simulink model "quad_control"  (Simulink 10.0)
settings: Solver=ode45  StartTime=0.0  StopTime=20  RelTol=1e-3  EnableMultiTasking=on
undefined symbols (not defined in the file): X, x, Y, Z
libraries: sm_lib x84, nesl_utility x46, simulink x30, fl_lib x4, sm_double_wishbone_suspension_lib x2, aerolibtransform2 x2, vrlib x1
(part 1 of 3)
settings Model: Creator=abdkadma  LastModifiedBy=bhisma
settings DataIOCC: LimitDataPoints=on
settings DebuggingCC: UnderspecifiedInitializationDetection=Simplified  MergeDetectMultiDrivingBlocksExec=error  SolverPrmCheckMsg=warning
settings GRTTargetCC: GeneratePreprocessorConditionals=Disable all  CombineOutputUpdateFcns=on  GRTInterface=off
settings ConfigComp: CovExternalEMLEnable=off
settings SimscapeCC: SimscapeNormalizeSystem=off
settings ConfigurationSet: Description=SimMechanics 2G

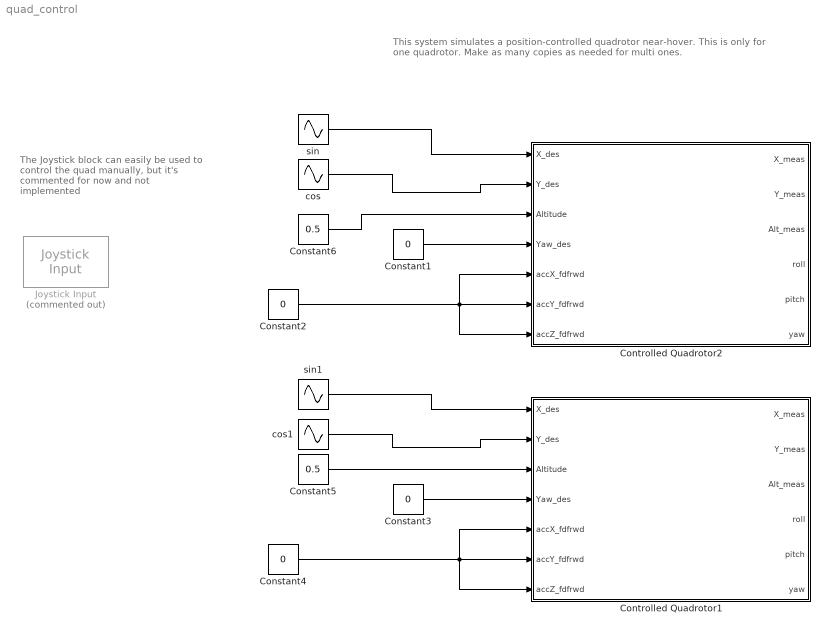
== system quad_control ==
  note: The Joystick block can easily
      | be used to control the quad manually,
      | but it's commented for now and
      | not implemented
  note: This system simulates a position-controlled quadrotor
      | near-hover. This is only for one quadrotor. Make as many copies as needed
      | for multi ones.
  Constant{1..4} (4 alike) : Constant  Value=0
  Constant5 : Constant  Value=0.5
  Constant6 : Constant  Value=0.5
  Controlled Quadrotor1 : Subsystem
      mask Display:
      | image('quadPic.jpg')
      | port_label('input',1,'x_des')
      | port_label('input',2,'y_des')
      | port_label('input',3,'Alt_des')
      | port_label('input',4,'Yaw_des')
      | port_label('input',5,'AccX_fedFwd')
      | port_label('input',6,'AccY_fedFwd')
      | port_label('input',7,'AccZ_fedFwd')
      | 
      | port_label('output',1,'x_meas')
      | port_label('output',2,'y_meas')
      | port_label('output',3,'z_meas')
      | port_label('output',4,'roll_meas')
      | port_label('output',5,'pitch_meas')
      | port_label('output',6,'yaw_meas')
  Controlled Quadrotor2 : Subsystem
      mask Display:
      | image('quadPic.jpg')
      | port_label('input',1,'x_des')
      | port_label('input',2,'y_des')
      | port_label('input',3,'Alt_des')
      | port_label('input',4,'Yaw_des')
      | port_label('input',5,'AccX_fedFwd')
      | port_label('input',6,'AccY_fedFwd')
      | port_label('input',7,'AccZ_fedFwd')
      | 
      | port_label('output',1,'x_meas')
      | port_label('output',2,'y_meas')
      | port_label('output',3,'z_meas')
      | port_label('output',4,'roll_meas')
      | port_label('output',5,'pitch_meas')
      | port_label('output',6,'yaw_meas')
  Joystick Input : vrlib/Joystick Input  Commented=on  joyid=1  adjustports=on  forcefeed=off
      settings: SourceProductName=Simulink
  cos : Sin  Amplitude=2  Phase=pi/2  SampleTime=0
  cos1 : Sin  SampleTime=0
  sin : Sin  Amplitude=2  SampleTime=0
  sin1 : Sin  Phase=pi/2  SampleTime=0
  wires:
  sin/1 -> Controlled Quadrotor2/1(X_des)
  cos/1 -> Controlled Quadrotor2/2(Y_des)
  Constant1/1 -> Controlled Quadrotor2/4(Yaw_des)
  Constant2/1 -> Controlled Quadrotor2/7(accZ_fdfrwd), Controlled Quadrotor2/5(accX_fdfrwd), Controlled Quadrotor2/6(accY_fdfrwd)
  Constant6/1 -> Controlled Quadrotor2/3(Altitude)
  sin1/1 -> Controlled Quadrotor1/1(X_des)
  cos1/1 -> Controlled Quadrotor1/2(Y_des)
  Constant3/1 -> Controlled Quadrotor1/4(Yaw_des)
  Constant4/1 -> Controlled Quadrotor1/7(accZ_fdfrwd), Controlled Quadrotor1/5(accX_fdfrwd), Controlled Quadrotor1/6(accY_fdfrwd)
  Constant5/1 -> Controlled Quadrotor1/3(Altitude)

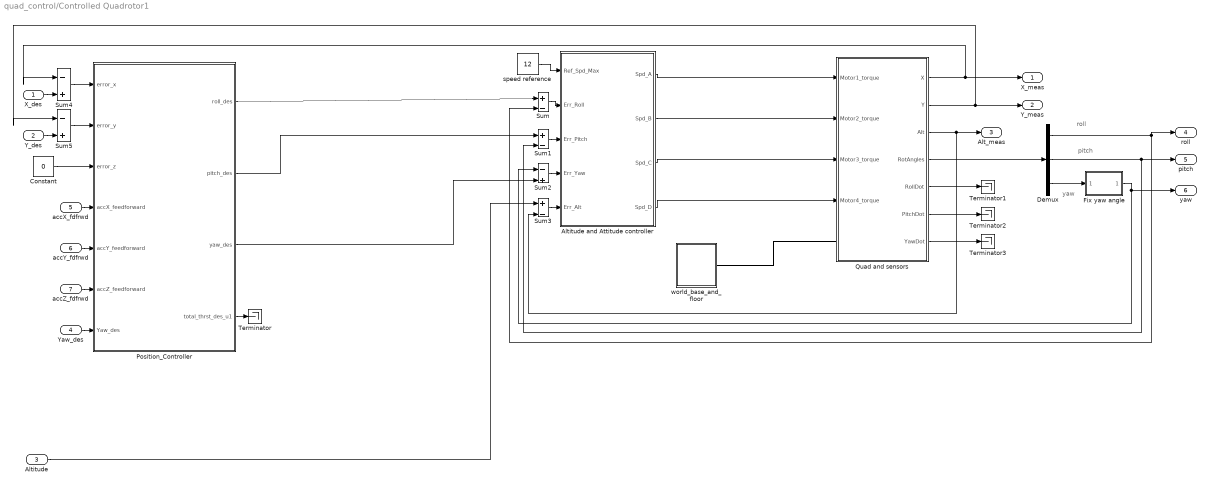
== system quad_control/Controlled Quadrotor1 ==
  note: yaw
  note: pitch
  note: roll
  X_des : Inport
  Y_des : Inport  Port=2
  Altitude : Inport  Port=3
  Yaw_des : Inport  Port=4
  accX_fdfrwd : Inport  Port=5
  accY_fdfrwd : Inport  Port=6
  accZ_fdfrwd : Inport  Port=7
  Altitude and Attitude controller : Subsystem
  Constant : Constant  Value=0
  Demux : Demux  Outputs=3
  Fix yaw angle : MATLAB Function  TreatAsAtomicUnit=on
  Position_Controller : Subsystem
  Quad and sensors : Subsystem
  Sum : Sum  Inputs=|+-
  Sum1 : Sum  Inputs=|+-
  Sum2 : Sum  Inputs=|-+
  Sum3 : Sum  Inputs=|+-
  Sum4 : Sum  Inputs=|-+
  Sum5 : Sum  Inputs=|-+
  Terminator{,1..3} (4 alike) : Terminator
  speed reference : Constant  Value=12
  world_base_and_floor : Subsystem
  X_meas : Outport
  Y_meas : Outport  Port=2
  Alt_meas : Outport  Port=3
  roll : Outport  Port=4
  pitch : Outport  Port=5
  yaw : Outport  Port=6
  wires:
  speed reference/1 -> Altitude and Attitude controller/1(Ref_Spd_Max)
  Sum1/1 -> Altitude and Attitude controller/3(Err_Pitch)
  Sum2/1 -> Altitude and Attitude controller/4(Err_Yaw)
  Sum3/1 -> Altitude and Attitude controller/5(Err_Alt)
  Altitude and Attitude controller/3(Spd_C) -> Quad and sensors/3(Motor3_torque)
  Altitude and Attitude controller/2(Spd_B) -> Quad and sensors/2(Motor2_torque)
  Altitude and Attitude controller/4(Spd_D) -> Quad and sensors/4(Motor4_torque)
  Altitude and Attitude controller/1(Spd_A) -> Quad and sensors/1(Motor1_torque)
  Demux/3 -> Fix yaw angle/1(yawangle)
  Position_Controller/3(yaw_des) -> Sum2/2
  Sum4/1 -> Position_Controller/1(error_x)
  Sum5/1 -> Position_Controller/2(error_y)
  Quad and sensors/1(X) -> X_meas/1, Sum4/1
  Position_Controller/1(roll_des) -> Sum/1
  Position_Controller/2(pitch_des) -> Sum1/1
  Sum/1 -> Altitude and Attitude controller/2(Err_Roll)
  accZ_fdfrwd/1 -> Position_Controller/6(accZ_feedforward)
  X_des/1 -> Sum4/2
  Altitude/1 -> Sum3/1
  Y_des/1 -> Sum5/2
  accY_fdfrwd/1 -> Position_Controller/5(accY_feedforward)
  accX_fdfrwd/1 -> Position_Controller/4(accX_feedforward)
  Position_Controller/4(total_thrst_des_u1) -> Terminator/1
  Constant/1 -> Position_Controller/3(error_z)
  Quad and sensors/5(RollDot) -> Terminator1/1
  Yaw_des/1 -> Position_Controller/7(Yaw_des)
  Quad and sensors/2(Y) -> Y_meas/1, Sum5/1
  Quad and sensors/3(Alt) -> Alt_meas/1, Sum3/2
  Quad and sensors/6(PitchDot) -> Terminator2/1
  Quad and sensors/7(YawDot) -> Terminator3/1
  Quad and sensors/4(RotAngles) -> Demux/1
  Fix yaw angle/1(anglefix) -> yaw/1, Sum2/1
  Demux/2 -> pitch/1, Sum1/2
  Demux/1 -> Sum/2, roll/1
  connections:
  world_base_and_floor/RConn1 -- Quad and sensors/LConn1

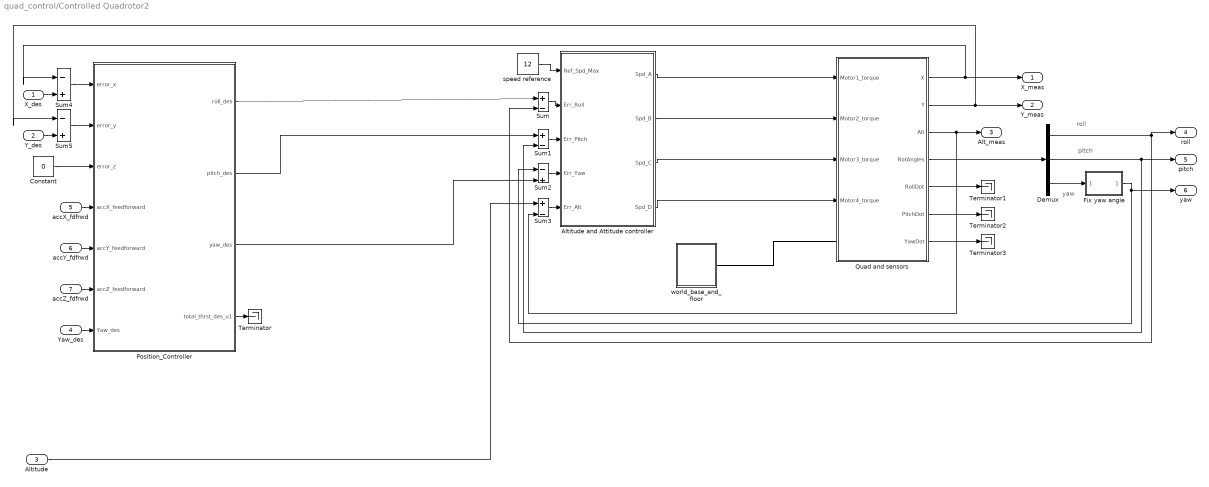
== system quad_control/Controlled Quadrotor2 ==
  note: yaw
  note: pitch
  note: roll
  X_des : Inport
  Y_des : Inport  Port=2
  Altitude : Inport  Port=3
  Yaw_des : Inport  Port=4
  accX_fdfrwd : Inport  Port=5
  accY_fdfrwd : Inport  Port=6
  accZ_fdfrwd : Inport  Port=7
  Altitude and Attitude controller : Subsystem
  Constant : Constant  Value=0
  Demux : Demux  Outputs=3
  Fix yaw angle : MATLAB Function  TreatAsAtomicUnit=on
  Position_Controller : Subsystem
  Quad and sensors : Subsystem
  Sum : Sum  Inputs=|+-
  Sum1 : Sum  Inputs=|+-
  Sum2 : Sum  Inputs=|-+
  Sum3 : Sum  Inputs=|+-
  Sum4 : Sum  Inputs=|-+
  Sum5 : Sum  Inputs=|-+
  Terminator{,1..3} (4 alike) : Terminator
  speed reference : Constant  Value=12
  world_base_and_floor : Subsystem
  X_meas : Outport
  Y_meas : Outport  Port=2
  Alt_meas : Outport  Port=3
  roll : Outport  Port=4
  pitch : Outport  Port=5
  yaw : Outport  Port=6
  wires:
  speed reference/1 -> Altitude and Attitude controller/1(Ref_Spd_Max)
  Sum1/1 -> Altitude and Attitude controller/3(Err_Pitch)
  Sum2/1 -> Altitude and Attitude controller/4(Err_Yaw)
  Sum3/1 -> Altitude and Attitude controller/5(Err_Alt)
  Altitude and Attitude controller/3(Spd_C) -> Quad and sensors/3(Motor3_torque)
  Altitude and Attitude controller/2(Spd_B) -> Quad and sensors/2(Motor2_torque)
  Altitude and Attitude controller/4(Spd_D) -> Quad and sensors/4(Motor4_torque)
  Altitude and Attitude controller/1(Spd_A) -> Quad and sensors/1(Motor1_torque)
  Demux/3 -> Fix yaw angle/1(yawangle)
  Position_Controller/3(yaw_des) -> Sum2/2
  Sum4/1 -> Position_Controller/1(error_x)
  Sum5/1 -> Position_Controller/2(error_y)
  Quad and sensors/1(X) -> X_meas/1, Sum4/1
  Position_Controller/1(roll_des) -> Sum/1
  Position_Controller/2(pitch_des) -> Sum1/1
  Sum/1 -> Altitude and Attitude controller/2(Err_Roll)
  accZ_fdfrwd/1 -> Position_Controller/6(accZ_feedforward)
  X_des/1 -> Sum4/2
  Altitude/1 -> Sum3/1
  Y_des/1 -> Sum5/2
  accY_fdfrwd/1 -> Position_Controller/5(accY_feedforward)
  accX_fdfrwd/1 -> Position_Controller/4(accX_feedforward)
  Position_Controller/4(total_thrst_des_u1) -> Terminator/1
  Constant/1 -> Position_Controller/3(error_z)
  Quad and sensors/5(RollDot) -> Terminator1/1
  Yaw_des/1 -> Position_Controller/7(Yaw_des)
  Quad and sensors/2(Y) -> Y_meas/1, Sum5/1
  Quad and sensors/3(Alt) -> Alt_meas/1, Sum3/2
  Quad and sensors/6(PitchDot) -> Terminator2/1
  Quad and sensors/7(YawDot) -> Terminator3/1
  Quad and sensors/4(RotAngles) -> Demux/1
  Fix yaw angle/1(anglefix) -> yaw/1, Sum2/1
  Demux/2 -> pitch/1, Sum1/2
  Demux/1 -> Sum/2, roll/1
  connections:
  world_base_and_floor/RConn1 -- Quad and sensors/LConn1

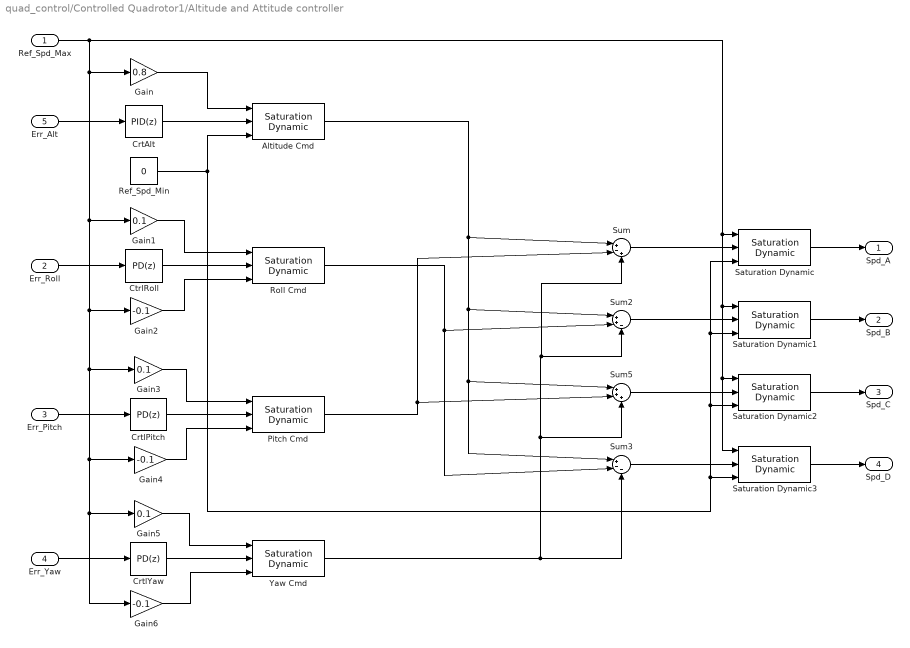
== system quad_control/Controlled Quadrotor1/Altitude and Attitude controller ==
  Ref_Spd_Max : Inport
  Err_Roll : Inport  Port=2
  Err_Pitch : Inport  Port=3
  Err_Yaw : Inport  Port=4
  Err_Alt : Inport  Port=5
  Altitude Cmd : simulink/Discontinuities/Saturation Dynamic  OutMin=[]  OutMax=[]  OutDataTypeStr=Inherit: Same as second input  OutDataType=fixdt(1, 16)  OutScaling=2^-10  DoSatur=off
  CrtAlt : simulink/Continuous/PID Controller  Controller=PID  TimeDomain=Discrete-time  SampleTime=0.001  IntegratorMethod=Forward Euler  FilterMethod=Forward Euler  Form=Parallel  P=20  I=10  D=5  N=100  InitialConditionSource=internal  InitialConditionForIntegrator=0  InitialConditionForFilter=0  ExternalReset=none  LimitOutput=off  UpperSaturationLimit=0.116  LowerSaturationLimit=-0.116  LinearizeAsGain=off  AntiWindupMode=none  Kb=1  TrackingMode=off  Kt=1  PParamMin=[]  PParamMax=[]  IParamMin=[]  IParamMax=[]  DParamMin=[]  DParamMax=[]  NParamMin=[]  NParamMax=[]  KbParamMin=[]  KbParamMax=[]  KtParamMin=[]  KtParamMax=[]  POutMin=[]  POutMax=[]  IOutMin=[]  IOutMax=[]  DOutMin=[]  DOutMax=[]  NOutMin=[]  NOutMax=[]  KbOutMin=[]  KbOutMax=[]  KtOutMin=[]  KtOutMax=[]  IntegratorOutMin=[]  IntegratorOutMax=[]  FilterOutMin=[]  FilterOutMax=[]  SumOutMin=[]  SumOutMax=[]  SumI1OutMin=[]  SumI1OutMax=[]  SumI2OutMin=[]  SumI2OutMax=[]  SumI3OutMin=[]  SumI3OutMax=[]  SumDOutMin=[]  SumDOutMax=[]  SaturationOutMin=[]  SaturationOutMax=[]  IntegratorContinuousStateAttributes=''  IntegratorStateMustResolveToSignalObject=off  IntegratorRTWStateStorageClass=Auto  FilterContinuousStateAttributes=''  FilterStateMustResolveToSignalObject=off  FilterRTWStateStorageClass=Auto  DifferentiatorICPrevScaledInput=0  DifferentiatorOutMin=[]  DifferentiatorOutMax=[]  UseFilter=on
  CrtlPitch : simulink/Continuous/PID Controller  Controller=PD  TimeDomain=Discrete-time  SampleTime=0.001  IntegratorMethod=Forward Euler  FilterMethod=Forward Euler  Form=Parallel  P=2  I=0  D=1  N=100  InitialConditionSource=internal  InitialConditionForIntegrator=0  InitialConditionForFilter=0  ExternalReset=none  LimitOutput=off  UpperSaturationLimit=+Inf  LowerSaturationLimit=0  LinearizeAsGain=off  AntiWindupMode=none  Kb=1  TrackingMode=off  Kt=1  PParamMin=[]  PParamMax=[]  IParamMin=[]  IParamMax=[]  DParamMin=[]  DParamMax=[]  NParamMin=[]  NParamMax=[]  KbParamMin=[]  KbParamMax=[]  KtParamMin=[]  KtParamMax=[]  POutMin=[]  POutMax=[]  IOutMin=[]  IOutMax=[]  DOutMin=[]  DOutMax=[]  NOutMin=[]  NOutMax=[]  KbOutMin=[]  KbOutMax=[]  KtOutMin=[]  KtOutMax=[]  IntegratorOutMin=[]  IntegratorOutMax=[]  FilterOutMin=[]  FilterOutMax=[]  SumOutMin=[]  SumOutMax=[]  SumI1OutMin=[]  SumI1OutMax=[]  SumI2OutMin=[]  SumI2OutMax=[]  SumI3OutMin=[]  SumI3OutMax=[]  SumDOutMin=[]  SumDOutMax=[]  SaturationOutMin=[]  SaturationOutMax=[]  IntegratorContinuousStateAttributes=''  IntegratorStateMustResolveToSignalObject=off  IntegratorRTWStateStorageClass=Auto  FilterContinuousStateAttributes=''  FilterStateMustResolveToSignalObject=off  FilterRTWStateStorageClass=Auto  DifferentiatorICPrevScaledInput=0  DifferentiatorOutMin=[]  DifferentiatorOutMax=[]  UseFilter=on
  CrtlYaw : simulink/Continuous/PID Controller  Controller=PD  TimeDomain=Discrete-time  SampleTime=0.001  IntegratorMethod=Forward Euler  FilterMethod=Forward Euler  Form=Parallel  P=0.05  I=1  D=0.01  N=100  InitialConditionSource=internal  InitialConditionForIntegrator=0  InitialConditionForFilter=0  ExternalReset=none  LimitOutput=off  UpperSaturationLimit=0.01  LowerSaturationLimit=-0.01  LinearizeAsGain=off  AntiWindupMode=none  Kb=1  TrackingMode=off  Kt=1  PParamMin=[]  PParamMax=[]  IParamMin=[]  IParamMax=[]  DParamMin=[]  DParamMax=[]  NParamMin=[]  NParamMax=[]  KbParamMin=[]  KbParamMax=[]  KtParamMin=[]  KtParamMax=[]  POutMin=[]  POutMax=[]  IOutMin=[]  IOutMax=[]  DOutMin=[]  DOutMax=[]  NOutMin=[]  NOutMax=[]  KbOutMin=[]  KbOutMax=[]  KtOutMin=[]  KtOutMax=[]  IntegratorOutMin=[]  IntegratorOutMax=[]  FilterOutMin=[]  FilterOutMax=[]  SumOutMin=[]  SumOutMax=[]  SumI1OutMin=[]  SumI1OutMax=[]  SumI2OutMin=[]  SumI2OutMax=[]  SumI3OutMin=[]  SumI3OutMax=[]  SumDOutMin=[]  SumDOutMax=[]  SaturationOutMin=[]  SaturationOutMax=[]  IntegratorContinuousStateAttributes=''  IntegratorStateMustResolveToSignalObject=off  IntegratorRTWStateStorageClass=Auto  FilterContinuousStateAttributes=''  FilterStateMustResolveToSignalObject=off  FilterRTWStateStorageClass=Auto  DifferentiatorICPrevScaledInput=0  DifferentiatorOutMin=[]  DifferentiatorOutMax=[]  UseFilter=on
  CtrlRoll : simulink/Continuous/PID Controller  Controller=PD  TimeDomain=Discrete-time  SampleTime=0.001  IntegratorMethod=Forward Euler  FilterMethod=Forward Euler  Form=Parallel  P=2  I=0  D=1  N=100  InitialConditionSource=internal  InitialConditionForIntegrator=0  InitialConditionForFilter=0  ExternalReset=none  LimitOutput=off  UpperSaturationLimit=+Inf  LowerSaturationLimit=0  LinearizeAsGain=off  AntiWindupMode=none  Kb=1  TrackingMode=off  Kt=1  PParamMin=[]  PParamMax=[]  IParamMin=[]  IParamMax=[]  DParamMin=[]  DParamMax=[]  NParamMin=[]  NParamMax=[]  KbParamMin=[]  KbParamMax=[]  KtParamMin=[]  KtParamMax=[]  POutMin=[]  POutMax=[]  IOutMin=[]  IOutMax=[]  DOutMin=[]  DOutMax=[]  NOutMin=[]  NOutMax=[]  KbOutMin=[]  KbOutMax=[]  KtOutMin=[]  KtOutMax=[]  IntegratorOutMin=[]  IntegratorOutMax=[]  FilterOutMin=[]  FilterOutMax=[]  SumOutMin=[]  SumOutMax=[]  SumI1OutMin=[]  SumI1OutMax=[]  SumI2OutMin=[]  SumI2OutMax=[]  SumI3OutMin=[]  SumI3OutMax=[]  SumDOutMin=[]  SumDOutMax=[]  SaturationOutMin=[]  SaturationOutMax=[]  IntegratorContinuousStateAttributes=''  IntegratorStateMustResolveToSignalObject=off  IntegratorRTWStateStorageClass=Auto  FilterContinuousStateAttributes=''  FilterStateMustResolveToSignalObject=off  FilterRTWStateStorageClass=Auto  DifferentiatorICPrevScaledInput=0  DifferentiatorOutMin=[]  DifferentiatorOutMax=[]  UseFilter=on
  Gain : Gain  Gain=0.8
  Gain1 : Gain  Gain=0.1
  Gain2 : Gain  Gain=-0.1
  Gain3 : Gain  Gain=0.1
  Gain4 : Gain  Gain=-0.1
  Gain5 : Gain  Gain=0.1
  Gain6 : Gain  Gain=-0.1
  Pitch Cmd : simulink/Discontinuities/Saturation Dynamic  OutMin=[]  OutMax=[]  OutDataTypeStr=Inherit: Same as second input  OutDataType=fixdt(1, 16)  OutScaling=2^-10  DoSatur=off
      settings: LockScale=on
  Ref_Spd_Min : Constant  Value=0
  Roll Cmd : simulink/Discontinuities/Saturation Dynamic  OutMin=[]  OutMax=[]  OutDataTypeStr=Inherit: Same as second input  OutDataType=fixdt(1, 16)  OutScaling=2^-10  DoSatur=off
      settings: LockScale=on
  Saturation Dynamic{,1..3} (4 alike) : simulink/Discontinuities/Saturation Dynamic  OutMin=[]  OutMax=[]  OutDataTypeStr=Inherit: Same as second input  OutDataType=fixdt(1, 16)  OutScaling=2^-10  DoSatur=off
  Sum : Sum  Inputs=|+-+
  Sum2 : Sum  Inputs=|++-
  Sum3 : Sum  Inputs=|+--
  Sum5 : Sum  Inputs=|+++
  Yaw Cmd : simulink/Discontinuities/Saturation Dynamic  OutMin=[]  OutMax=[]  OutDataTypeStr=Inherit: Same as second input  OutDataType=fixdt(1, 16)  OutScaling=2^-10  DoSatur=off
      settings: LockScale=on
  Spd_A : Outport
  Spd_B : Outport  Port=2
  Spd_C : Outport  Port=3
  Spd_D : Outport  Port=4
  wires:
  Saturation Dynamic/1 -> Spd_A/1
  Saturation Dynamic1/1 -> Spd_B/1
  Saturation Dynamic2/1 -> Spd_C/1
  Saturation Dynamic3/1 -> Spd_D/1
  Sum/1 -> Saturation Dynamic/2
  Sum2/1 -> Saturation Dynamic1/2
  Sum5/1 -> Saturation Dynamic2/2
  Sum3/1 -> Saturation Dynamic3/2
  Ref_Spd_Max/1 -> Gain3/1, Gain4/1, Gain5/1, Gain6/1, Gain2/1, Gain1/1, Gain/1, Saturation Dynamic3/1, Saturation Dynamic2/1, Saturation Dynamic1/1, Saturation Dynamic/1
  Ref_Spd_Min/1 -> Saturation Dynamic/3, Saturation Dynamic1/3, Saturation Dynamic2/3, Saturation Dynamic3/3, Altitude Cmd/3
  Err_Alt/1 -> CrtAlt/1
  CrtAlt/1 -> Altitude Cmd/2
  Altitude Cmd/1 -> Sum3/1, Sum5/1, Sum2/1, Sum/1
  Err_Roll/1 -> CtrlRoll/1
  Gain/1 -> Altitude Cmd/1
  CtrlRoll/1 -> Roll Cmd/2
  Gain2/1 -> Roll Cmd/3
  Gain1/1 -> Roll Cmd/1
  Roll Cmd/1 -> Sum2/2, Sum3/2
  Err_Pitch/1 -> CrtlPitch/1
  CrtlPitch/1 -> Pitch Cmd/2
  Gain3/1 -> Pitch Cmd/1
  Gain4/1 -> Pitch Cmd/3
  Pitch Cmd/1 -> Sum/2, Sum5/2
  Err_Yaw/1 -> CrtlYaw/1
  CrtlYaw/1 -> Yaw Cmd/2
  Gain5/1 -> Yaw Cmd/1
  Gain6/1 -> Yaw Cmd/3
  Yaw Cmd/1 -> Sum/3, Sum2/3, Sum5/3, Sum3/3

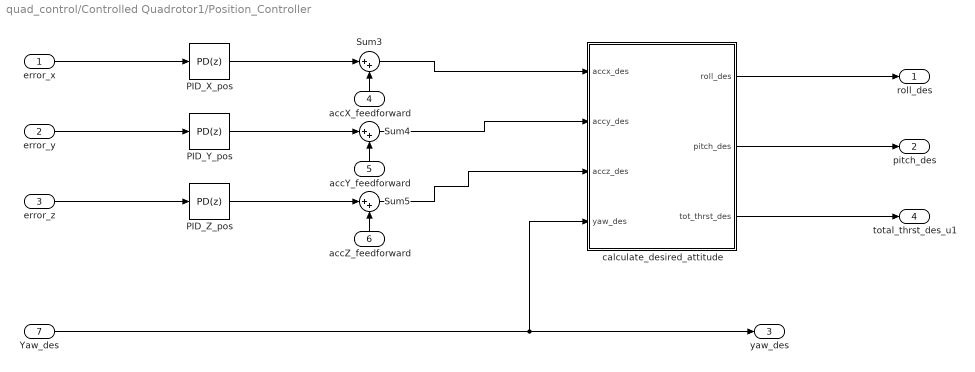
== system quad_control/Controlled Quadrotor1/Position_Controller ==
  error_x : Inport
  error_y : Inport  Port=2
  error_z : Inport  Port=3
  accX_feedforward : Inport  Port=4
  accY_feedforward : Inport  Port=5
  accZ_feedforward : Inport  Port=6
  Yaw_des : Inport  Port=7
  PID_X_pos : simulink/Continuous/PID Controller  Controller=PD  TimeDomain=Discrete-time  SampleTime=0.01  IntegratorMethod=Forward Euler  FilterMethod=Forward Euler  Form=Parallel  P=10  I=1  D=3  N=148.847847480226  InitialConditionSource=internal  InitialConditionForIntegrator=0  InitialConditionForFilter=0  ExternalReset=none  LimitOutput=off  UpperSaturationLimit=inf  LowerSaturationLimit=-inf  LinearizeAsGain=on  AntiWindupMode=none  Kb=1  TrackingMode=off  Kt=1  PParamMin=[]  PParamMax=[]  IParamMin=[]  IParamMax=[]  DParamMin=[]  DParamMax=[]  NParamMin=[]  NParamMax=[]  KbParamMin=[]  KbParamMax=[]  KtParamMin=[]  KtParamMax=[]  POutMin=[]  POutMax=[]  IOutMin=[]  IOutMax=[]  DOutMin=[]  DOutMax=[]  NOutMin=[]  NOutMax=[]  KbOutMin=[]  KbOutMax=[]  KtOutMin=[]  KtOutMax=[]  IntegratorOutMin=[]  IntegratorOutMax=[]  FilterOutMin=[]  FilterOutMax=[]  SumOutMin=[]  SumOutMax=[]  SumI1OutMin=[]  SumI1OutMax=[]  SumI2OutMin=[]  SumI2OutMax=[]  SumI3OutMin=[]  SumI3OutMax=[]  SumDOutMin=[]  SumDOutMax=[]  SaturationOutMin=[]  SaturationOutMax=[]  IntegratorContinuousStateAttributes=''  IntegratorStateMustResolveToSignalObject=off  IntegratorRTWStateStorageClass=Auto  FilterContinuousStateAttributes=''  FilterStateMustResolveToSignalObject=off  FilterRTWStateStorageClass=Auto  DifferentiatorICPrevScaledInput=0  DifferentiatorOutMin=[]  DifferentiatorOutMax=[]  UseFilter=on
  PID_Y_pos : simulink/Continuous/PID Controller  Controller=PD  TimeDomain=Discrete-time  SampleTime=0.01  IntegratorMethod=Forward Euler  FilterMethod=Forward Euler  Form=Parallel  P=10  I=1  D=3  N=100  InitialConditionSource=internal  InitialConditionForIntegrator=0  InitialConditionForFilter=0  ExternalReset=none  LimitOutput=off  UpperSaturationLimit=inf  LowerSaturationLimit=-inf  LinearizeAsGain=on  AntiWindupMode=none  Kb=1  TrackingMode=off  Kt=1  PParamMin=[]  PParamMax=[]  IParamMin=[]  IParamMax=[]  DParamMin=[]  DParamMax=[]  NParamMin=[]  NParamMax=[]  KbParamMin=[]  KbParamMax=[]  KtParamMin=[]  KtParamMax=[]  POutMin=[]  POutMax=[]  IOutMin=[]  IOutMax=[]  DOutMin=[]  DOutMax=[]  NOutMin=[]  NOutMax=[]  KbOutMin=[]  KbOutMax=[]  KtOutMin=[]  KtOutMax=[]  IntegratorOutMin=[]  IntegratorOutMax=[]  FilterOutMin=[]  FilterOutMax=[]  SumOutMin=[]  SumOutMax=[]  SumI1OutMin=[]  SumI1OutMax=[]  SumI2OutMin=[]  SumI2OutMax=[]  SumI3OutMin=[]  SumI3OutMax=[]  SumDOutMin=[]  SumDOutMax=[]  SaturationOutMin=[]  SaturationOutMax=[]  IntegratorContinuousStateAttributes=''  IntegratorStateMustResolveToSignalObject=off  IntegratorRTWStateStorageClass=Auto  FilterContinuousStateAttributes=''  FilterStateMustResolveToSignalObject=off  FilterRTWStateStorageClass=Auto  DifferentiatorICPrevScaledInput=0  DifferentiatorOutMin=[]  DifferentiatorOutMax=[]  UseFilter=on
  PID_Z_pos : simulink/Continuous/PID Controller  Controller=PD  TimeDomain=Discrete-time  SampleTime=0.01  IntegratorMethod=Forward Euler  FilterMethod=Forward Euler  Form=Parallel  P=2  I=10  D=0.001  N=100  InitialConditionSource=internal  InitialConditionForIntegrator=0  InitialConditionForFilter=0  ExternalReset=none  LimitOutput=off  UpperSaturationLimit=inf  LowerSaturationLimit=-inf  LinearizeAsGain=on  AntiWindupMode=none  Kb=1  TrackingMode=off  Kt=1  PParamMin=[]  PParamMax=[]  IParamMin=[]  IParamMax=[]  DParamMin=[]  DParamMax=[]  NParamMin=[]  NParamMax=[]  KbParamMin=[]  KbParamMax=[]  KtParamMin=[]  KtParamMax=[]  POutMin=[]  POutMax=[]  IOutMin=[]  IOutMax=[]  DOutMin=[]  DOutMax=[]  NOutMin=[]  NOutMax=[]  KbOutMin=[]  KbOutMax=[]  KtOutMin=[]  KtOutMax=[]  IntegratorOutMin=[]  IntegratorOutMax=[]  FilterOutMin=[]  FilterOutMax=[]  SumOutMin=[]  SumOutMax=[]  SumI1OutMin=[]  SumI1OutMax=[]  SumI2OutMin=[]  SumI2OutMax=[]  SumI3OutMin=[]  SumI3OutMax=[]  SumDOutMin=[]  SumDOutMax=[]  SaturationOutMin=[]  SaturationOutMax=[]  IntegratorContinuousStateAttributes=''  IntegratorStateMustResolveToSignalObject=off  IntegratorRTWStateStorageClass=Auto  FilterContinuousStateAttributes=''  FilterStateMustResolveToSignalObject=off  FilterRTWStateStorageClass=Auto  DifferentiatorICPrevScaledInput=0  DifferentiatorOutMin=[]  DifferentiatorOutMax=[]  UseFilter=on
  Sum3 : Sum  Inputs=|++
  Sum4 : Sum  Inputs=|++
  Sum5 : Sum  Inputs=|++
  calculate_desired_attitude : MATLAB Function  TreatAsAtomicUnit=on
  roll_des : Outport
  pitch_des : Outport  Port=2
  yaw_des : Outport  Port=3
  total_thrst_des_u1 : Outport  Port=4
  wires:
  PID_Z_pos/1 -> Sum5/1
  PID_Y_pos/1 -> Sum4/1
  accX_feedforward/1 -> Sum3/2
  calculate_desired_attitude/3(tot_thrst_des) -> total_thrst_des_u1/1
  Yaw_des/1 -> calculate_desired_attitude/4(yaw_des), yaw_des/1
  accZ_feedforward/1 -> Sum5/2
  accY_feedforward/1 -> Sum4/2
  Sum4/1 -> calculate_desired_attitude/2(accy_des)
  Sum3/1 -> calculate_desired_attitude/1(accx_des)
  PID_X_pos/1 -> Sum3/1
  Sum5/1 -> calculate_desired_attitude/3(accz_des)
  error_x/1 -> PID_X_pos/1
  error_y/1 -> PID_Y_pos/1
  error_z/1 -> PID_Z_pos/1
  calculate_desired_attitude/1(roll_des) -> roll_des/1
  calculate_desired_attitude/2(pitch_des) -> pitch_des/1

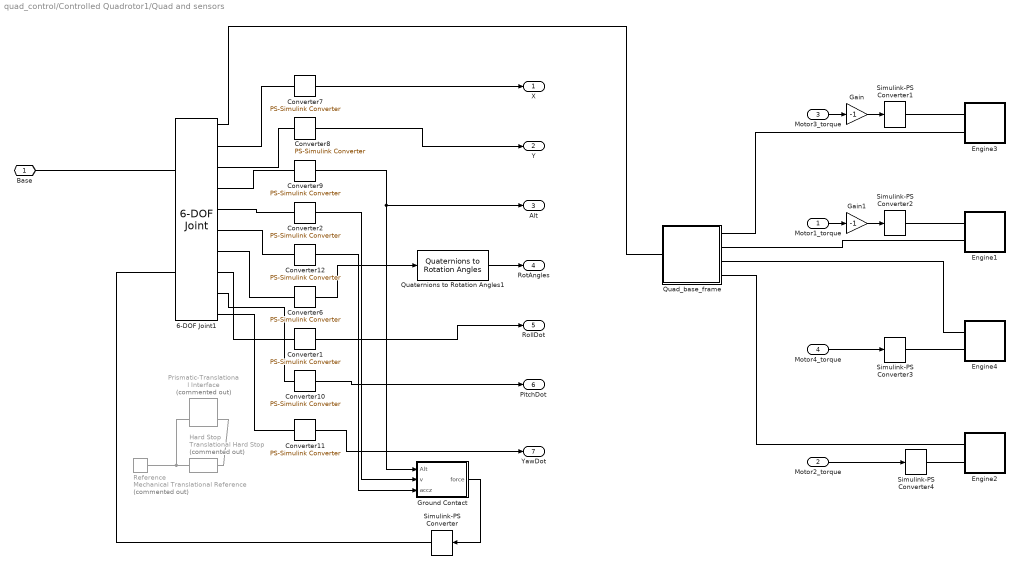
== system quad_control/Controlled Quadrotor1/Quad and sensors ==
  Motor1_torque : Inport
  Motor2_torque : Inport  Port=2
  Motor3_torque : Inport  Port=3
  Motor4_torque : Inport  Port=4
  6-DOF Joint1 : sm_lib/Joints/6-DOF Joint  SenseConstraintForce=off  SenseConstraintForceX=off  SenseConstraintForceY=off  SenseConstraintForceZ=off  SenseConstraintTorque=off  SenseConstraintTorqueX=off  SenseConstraintTorqueY=off  SenseConstraintTorqueZ=off  SenseTotalForce=off  SenseTotalForceX=off  SenseTotalForceY=off  SenseTotalForceZ=off  SenseTotalTorque=off  SenseTotalTorqueX=off  SenseTotalTorqueY=off  SenseTotalTorqueZ=off  CompositeWrenchDir=FollowerOnBase  CompositeWrenchFrame=BaseFrame  PxEquilibriumPosition=0  PxEquilibriumPositionUnits=m  PxSpringStiffness=0  PxSpringStiffnessUnits=N/m  PxDampingCoefficient=0  PxDampingCoefficientUnits=N/(m/s)  PxTorqueActuationMode=NoTorque  PxMotionActuationMode=ComputedMotion  PxSensePosition=on  PxSenseVelocity=off  PxSenseAcceleration=off  PxSenseTorqueForce=off  PxPositionTargetValue=1  PxPositionTargetValueUnits=m  PxPositionTargetSpecify=off  PxPositionTargetPriority=High  PxVelocityTargetValue=0  PxVelocityTargetValueUnits=m/s  PxVelocityTargetSpecify=off  PxVelocityTargetPriority=High  PyEquilibriumPosition=0  PyEquilibriumPositionUnits=m  PySpringStiffness=0  PySpringStiffnessUnits=N/m  PyDampingCoefficient=0  PyDampingCoefficientUnits=N/(m/s)  PyTorqueActuationMode=NoTorque  PyMotionActuationMode=ComputedMotion  PySensePosition=on  PySenseVelocity=off  PySenseAcceleration=off  PySenseTorqueForce=off  PyPositionTargetValue=0  PyPositionTargetValueUnits=m  PyPositionTargetSpecify=off  PyPositionTargetPriority=High  PyVelocityTargetValue=0  PyVelocityTargetValueUnits=m/s  PyVelocityTargetSpecify=off  PyVelocityTargetPriority=High  PzEquilibriumPosition=0  PzEquilibriumPositionUnits=m  PzSpringStiffness=0  PzSpringStiffnessUnits=N/m  PzDampingCoefficient=0  PzDampingCoefficientUnits=N/(m/s)  PzTorqueActuationMode=InputTorque  PzMotionActuationMode=ComputedMotion  PzSensePosition=on  PzSenseVelocity=on  PzSenseAcceleration=on  PzSenseTorqueForce=off  PzPositionTargetValue=2  PzPositionTargetValueUnits=m  PzPositionTargetSpecify=off  PzPositionTargetPriority=High  PzVelocityTargetValue=0  PzVelocityTargetValueUnits=m/s  PzVelocityTargetSpecify=off  PzVelocityTargetPriority=High  SphDefPosRotationMethod=None  SphDefPosRotationAngleUnits=deg  SphDefPosRotationStandardAxis=+Z  SphDefPosRotationAngle=0.0  SphDefPosRotationArbitraryAxis=[0 0 1]  SphDefPosFollAlignAxisA=+X  SphDefPosBaseAlignAxisA=+Y  SphDefPosFollAlignAxisB=+Y  SphDefPosBaseAlignAxisB=+Z  SphDefPosRotationMatrix=[1 0 0; 0 1 0; 0 0 1]  SphEqPosRotationMethod=None  SphEqPosRotationAngleUnits=deg  SphEqPosRotationStandardAxis=+Z  SphEqPosRotationAngle=0.0  SphEqPosRotationArbitraryAxis=[0 0 1]  SphEqPosFollAlignAxisA=+X  SphEqPosBaseAlignAxisA=+Y  SphEqPosFollAlignAxisB=+Y  SphEqPosBaseAlignAxisB=+Z  SphEqPosRotationMatrix=[1 0 0; 0 1 0; 0 0 1]  SphSpringStiffness=0  SphSpringStiffnessUnits=N*m/deg  SphDampingCoefficient=0  SphDampingCoefficientUnits=N*m/(deg/s)  SphActuateTorqueX=off  SphActuateTorqueY=off  SphActuateTorqueZ=off  SphActuateTorque=off  SphTorqueActuationMode=NoTorque  SphMotionActuationMode=ComputedMotion  SphActuationFrame=BaseFrame  SphSensePosition=on  SphSenseVelocityX=on  SphSenseVelocityY=on  SphSenseVelocityZ=on  SphSenseVelocity=off  SphSenseAccelerationX=off  SphSenseAccelerationY=off  SphSenseAccelerationZ=off  SphSenseAcceleration=off  SphSenseTorqueX=off  SphSenseTorqueY=off  SphSenseTorqueZ=off  SphSenseTorqueForce=off  SphSensingFrame=BaseFrame  SphPositionTargetRotationMethod=None  SphPositionTargetRotationAngleUnits=deg  SphPositionTargetRotationStandardAxis=+Z  SphPositionTargetRotationAngle=0.0  SphPositionTargetRotationArbitraryAxis=[0 0 1]  SphPositionTargetFollAlignAxisA=+X  SphPositionTargetBaseAlignAxisA=+Y  SphPositionTargetFollAlignAxisB=+Y  SphPositionTargetBaseAlignAxisB=+Z  SphPositionTargetRotationMatrix=[1 0 0; 0 1 0; 0 0 1]  SphPositionTargetSpecify=off  SphPositionTargetPriority=High  SphVelocityTargetValue=[0 0 0]  SphVelocityTargetValueUnits=deg/s  SphVelocityTargetSpecify=off  SphVelocityTargetPriority=High  SphVelocityTargetInFollowerFrame=on  BlockFunction=simmechanics.library.joints.sixdof_joint
  Converter{1..2,6..12} (9 alike) : nesl_utility/PS-Simulink Converter  PhysicalDomain=network_engine_domain  SubClassName=ps_output  LeftPortType=input  RightPortType=output  PseudoPeriodic=off  Frequencies=[]  Unit=1  AffineConversion=off
  Engine1 : Subsystem
  Engine2 : Subsystem
  Engine3 : Subsystem
  Engine4 : Subsystem
  Gain : Gain  Gain=-1
  Gain1 : Gain  Gain=-1
  Ground Contact : MATLAB Function  TreatAsAtomicUnit=on
  Hard Stop : fl_lib/Mechanical/Translational Elements/Translational Hard Stop  Commented=on  upper_bnd=6 m  lower_bnd=-x m  stiff_up=2e6 N/m  stiff_low=2e6 N/m  D_up=150 N/(m/s)  D_low=150 N/(m/s)  v_specify=off  v_priority=High  v=0 m/s  f_specify=off  f_priority=High  f=0 N  x_specify=on  x_priority=High  x=1 cm
  Prismatic-Translational Interface : sm_double_wishbone_suspension_lib/Testing Platform/Prismatic-Translational Interface  Commented=on
  Quad_base_frame : Subsystem
  Quaternions to Rotation Angles1 : aerolibtransform2/Quaternions to Rotation Angles  rotationOrder=XYZ
      settings: SourceProductName=Aerospace Blockset  SourceProductBaseCode=AE
  Reference : fl_lib/Mechanical/Translational Elements/Mechanical Translational Reference  Commented=on
  Simulink-PS Converter{,1..4} (5 alike) : nesl_utility/Simulink-PS Converter  PhysicalDomain=network_engine_domain  SubClassName=ps_input  LeftPortType=input  RightPortType=output  PseudoPeriodic=off  Frequencies=[]  NoiseDistribution=none  NoiseParameters=[]  Unit=1  AffineConversion=off  InputFiltering=off  SimscapeFilterOrder=1  InputFilterTimeConstant=0.001  UdotUserProvided=1
  Base : PMIOPort  Side=Left
  X : Outport
  Y : Outport  Port=2
  Alt : Outport  Port=3
  RotAngles : Outport  Port=4
  RollDot : Outport  Port=5
  PitchDot : Outport  Port=6
  YawDot : Outport  Port=7
  wires:
  Converter6/1 -> Quaternions to Rotation Angles1/1
  Quaternions to Rotation Angles1/1 -> RotAngles/1
  Converter7/1 -> X/1
  Converter8/1 -> Y/1
  Converter1/1 -> RollDot/1
  Converter10/1 -> PitchDot/1
  Converter11/1 -> YawDot/1
  Converter9/1 -> Alt/1, Ground Contact/1(Alt)
  Converter2/1 -> Ground Contact/2(v)
  Ground Contact/1(force) -> Simulink-PS Converter/1
  Converter12/1 -> Ground Contact/3(accz)
  Motor3_torque/1 -> Gain/1
  Motor1_torque/1 -> Gain1/1
  Motor4_torque/1 -> Simulink-PS Converter3/1
  Motor2_torque/1 -> Simulink-PS Converter4/1
  Gain/1 -> Simulink-PS Converter1/1
  Gain1/1 -> Simulink-PS Converter2/1
  connections:
  6-DOF Joint1/RConn1 -- Quad_base_frame/LConn1
  6-DOF Joint1/LConn1 -- Base/RConn1
  Converter8/LConn1 -- 6-DOF Joint1/RConn3
  Converter7/LConn1 -- 6-DOF Joint1/RConn2
  Converter9/LConn1 -- 6-DOF Joint1/RConn4
  Hard Stop/RConn1 -- Prismatic-Translational Interface/RConn2 -- Reference/LConn1
  Prismatic-Translational Interface/LConn2 -- Hard Stop/LConn1
  Converter2/LConn1 -- 6-DOF Joint1/RConn5
  6-DOF Joint1/RConn7 -- Converter6/LConn1
  6-DOF Joint1/RConn8 -- Converter1/LConn1
  6-DOF Joint1/RConn9 -- Converter10/LConn1
  6-DOF Joint1/RConn10 -- Converter11/LConn1
  Converter12/LConn1 -- 6-DOF Joint1/RConn6
  Engine3/LConn2 -- Quad_base_frame/RConn1
  Engine1/LConn2 -- Quad_base_frame/RConn2
  Engine4/LConn1 -- Quad_base_frame/RConn3
  Engine2/LConn1 -- Quad_base_frame/RConn4
  Simulink-PS Converter1/RConn1 -- Engine3/LConn1
  Simulink-PS Converter2/RConn1 -- Engine1/LConn1
  Simulink-PS Converter3/RConn1 -- Engine4/LConn2
  Simulink-PS Converter4/RConn1 -- Engine2/LConn2
  Simulink-PS Converter/RConn1 -- 6-DOF Joint1/LConn2

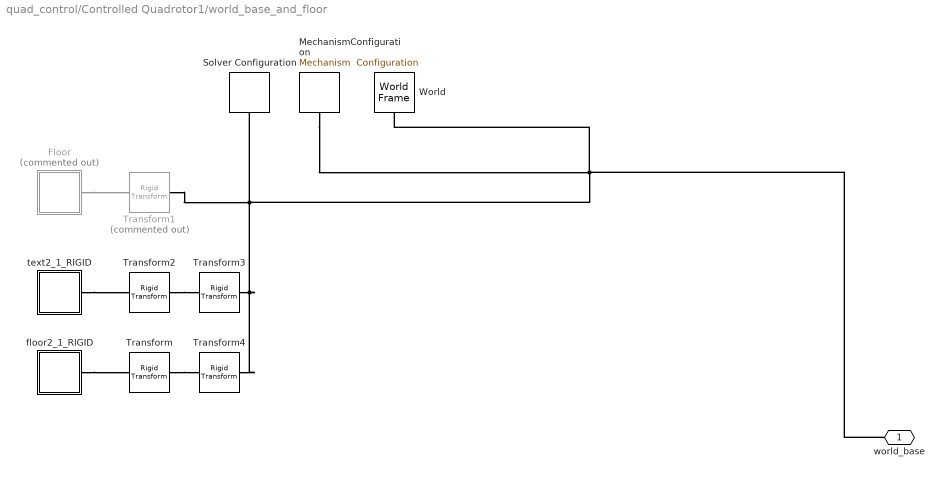
== system quad_control/Controlled Quadrotor1/world_base_and_floor ==
  Floor : Subsystem  Commented=on
  MechanismConfiguration : sm_lib/Utilities/Mechanism  Configuration  GravityVector=[0 0 -9.8]  GravityUnits=m/s^2  LinearizationDelta=0.001  BlockFunction=simmechanics.library.utilities.mechanism_configuration
      settings: SourceProductName=Simscape Multibody  SourceProductBaseCode=MS
  Solver Configuration : nesl_utility/Solver Configuration  PhysicalDomain=network_engine_domain  SubClassName=solver  LeftPortType=input  RightPortType=generic  Accelerate=off  Tones=[]  Harmonics=[]  SimulateNoise=off  Profile=off  UseLocalSampling=off  EnableSwitchedLinearOptims=on  FrequencyDomain=off  UseCCode=off  RelTol=0.001  AbsTol=1e-06  MinStep=1e-09  ToWorkspace=off  DoDC=off  ResidualTolerance=1e-09  UseLocalSolver=off  LocalSolverChoice=NE_BACKWARD_EULER_ADVANCER  LocalSolverSampleTime=0.001  DoFixedCost=off  MaxNonlinIter=3  MaxModeIter=2  LinearAlgebra=Sparse  DelaysMemoryBudget=1024  AutomaticFiltering=on  FilteringTimeConstant=0.001
  Transform : sm_lib/Frames and  Transforms/Rigid  Transform  TranslationMethod=Cartesian  TranslationLengthUnit=m  TranslationStandardAxis=+Z  TranslationStandardOffset=0  TranslationCartesianOffset=[-0.070528024651366206 0.0095986732478654524 -0.019304519570755498]  TranslationROffset=0  TranslationROffsetUnits=m  TranslationZOffset=0  TranslationZOffsetUnits=m  TranslationThetaOffset=0  TranslationThetaOffsetUnits=deg  RotationMethod=None  RotationAngleUnits=deg  RotationStandardAxis=+Z  RotationAngle=0.0  RotationArbitraryAxis=[0 0 1]  FollAlignAxisA=+X  BaseAlignAxisA=+Y  FollAlignAxisB=+Y  BaseAlignAxisB=+Z  RotationMatrix=[1 0 0; 0 1 0; 0 0 1]  BlockFunction=simmechanics.library.frames_transforms.rigid_transform
      settings: SourceProductName=Simscape Multibody  SourceProductBaseCode=MS
  Transform1 : sm_lib/Frames and  Transforms/Rigid  Transform  Commented=on  TranslationMethod=StandardAxis  TranslationLengthUnit=cm  TranslationStandardAxis=-Z  TranslationStandardOffset=15  TranslationCartesianOffset=[-0.044970866630080319 0.021117081145462624 -0.04061611986513753]  TranslationROffset=0  TranslationROffsetUnits=m  TranslationZOffset=0  TranslationZOffsetUnits=m  TranslationThetaOffset=0  TranslationThetaOffsetUnits=deg  RotationMethod=None  RotationAngleUnits=deg  RotationStandardAxis=+Z  RotationAngle=0.0  RotationArbitraryAxis=[0 0 1]  FollAlignAxisA=+X  BaseAlignAxisA=+Y  FollAlignAxisB=+Y  BaseAlignAxisB=+Z  RotationMatrix=[1 0 0; 0 1 0; 0 0 1]  BlockFunction=simmechanics.library.frames_transforms.rigid_transform
      settings: SourceProductName=Simscape Multibody  SourceProductBaseCode=MS
  Transform2 : sm_lib/Frames and  Transforms/Rigid  Transform  TranslationMethod=Cartesian  TranslationLengthUnit=m  TranslationStandardAxis=+Z  TranslationStandardOffset=0  TranslationCartesianOffset=[-0.029524654807930706 -2.1191477586035332 0.080695480429244501]  TranslationROffset=0  TranslationROffsetUnits=m  TranslationZOffset=0  TranslationZOffsetUnits=m  TranslationThetaOffset=0  TranslationThetaOffsetUnits=deg  RotationMethod=None  RotationAngleUnits=deg  RotationStandardAxis=+Z  RotationAngle=0.0  RotationArbitraryAxis=[0 0 1]  FollAlignAxisA=+X  BaseAlignAxisA=+Y  FollAlignAxisB=+Y  BaseAlignAxisB=+Z  RotationMatrix=[1 0 0; 0 1 0; 0 0 1]  BlockFunction=simmechanics.library.frames_transforms.rigid_transform
      settings: SourceProductName=Simscape Multibody  SourceProductBaseCode=MS
  Transform3 : sm_lib/Frames and  Transforms/Rigid  Transform  TranslationMethod=StandardAxis  TranslationLengthUnit=cm  TranslationStandardAxis=-Z  TranslationStandardOffset=15  TranslationCartesianOffset=[-0.029524654807930706 -2.1191477586035332 0.080695480429244501]  TranslationROffset=0  TranslationROffsetUnits=m  TranslationZOffset=0  TranslationZOffsetUnits=m  TranslationThetaOffset=0  TranslationThetaOffsetUnits=deg  RotationMethod=None  RotationAngleUnits=deg  RotationStandardAxis=+Z  RotationAngle=0.0  RotationArbitraryAxis=[0 0 1]  FollAlignAxisA=+X  BaseAlignAxisA=+Y  FollAlignAxisB=+Y  BaseAlignAxisB=+Z  RotationMatrix=[1 0 0; 0 1 0; 0 0 1]  BlockFunction=simmechanics.library.frames_transforms.rigid_transform
      settings: SourceProductName=Simscape Multibody  SourceProductBaseCode=MS
  Transform4 : sm_lib/Frames and  Transforms/Rigid  Transform  TranslationMethod=StandardAxis  TranslationLengthUnit=cm  TranslationStandardAxis=-Z  TranslationStandardOffset=15  TranslationCartesianOffset=[-0.070528024651366206 0.0095986732478654524 -0.019304519570755498]  TranslationROffset=0  TranslationROffsetUnits=m  TranslationZOffset=0  TranslationZOffsetUnits=m  TranslationThetaOffset=0  TranslationThetaOffsetUnits=deg  RotationMethod=None  RotationAngleUnits=deg  RotationStandardAxis=+Z  RotationAngle=0.0  RotationArbitraryAxis=[0 0 1]  FollAlignAxisA=+X  BaseAlignAxisA=+Y  FollAlignAxisB=+Y  BaseAlignAxisB=+Z  RotationMatrix=[1 0 0; 0 1 0; 0 0 1]  BlockFunction=simmechanics.library.frames_transforms.rigid_transform
      settings: SourceProductName=Simscape Multibody  SourceProductBaseCode=MS
  World : sm_lib/Frames and  Transforms/World Frame  BlockFunction=simmechanics.library.frames_transforms.world_frame
      settings: SourceProductName=Simscape Multibody  SourceProductBaseCode=MS
  floor2_1_RIGID : Subsystem
  text2_1_RIGID : Subsystem
  world_base : PMIOPort  Side=Right
  connections:
  Transform3/LConn1 -- Transform1/LConn1 -- Solver Configuration/RConn1 -- MechanismConfiguration/RConn1 -- World/RConn1 -- world_base/RConn1 -- Transform4/LConn1
  Floor/LConn1 -- Transform1/RConn1
  text2_1_RIGID/LConn1 -- Transform2/RConn1
  floor2_1_RIGID/LConn1 -- Transform/RConn1
  Transform2/LConn1 -- Transform3/RConn1
  Transform/LConn1 -- Transform4/RConn1

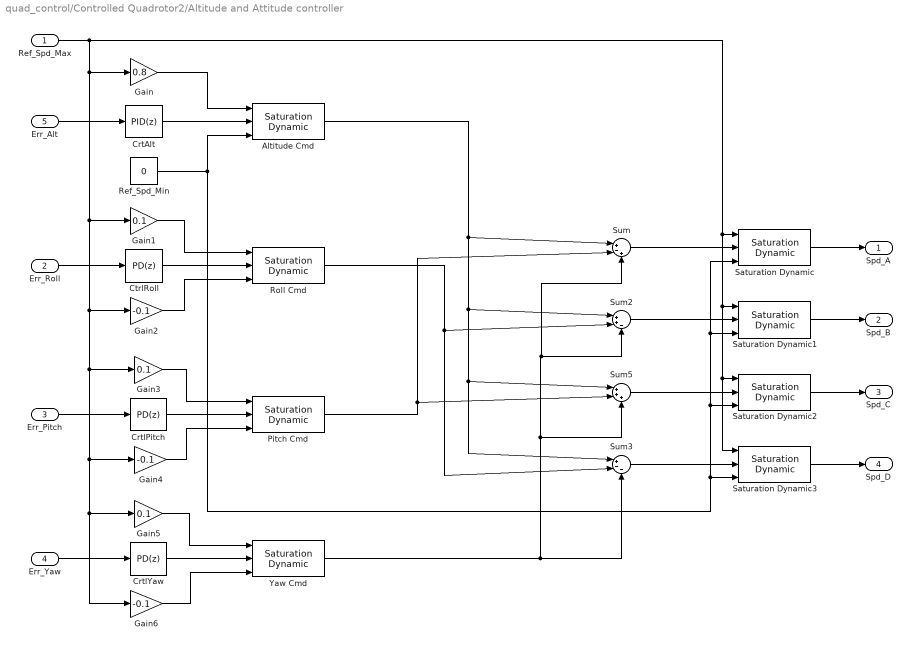
== system quad_control/Controlled Quadrotor2/Altitude and Attitude controller ==
  Ref_Spd_Max : Inport
  Err_Roll : Inport  Port=2
  Err_Pitch : Inport  Port=3
  Err_Yaw : Inport  Port=4
  Err_Alt : Inport  Port=5
  Altitude Cmd : simulink/Discontinuities/Saturation Dynamic  OutMin=[]  OutMax=[]  OutDataTypeStr=Inherit: Same as second input  OutDataType=fixdt(1, 16)  OutScaling=2^-10  DoSatur=off
  CrtAlt : simulink/Continuous/PID Controller  Controller=PID  TimeDomain=Discrete-time  SampleTime=0.001  IntegratorMethod=Forward Euler  FilterMethod=Forward Euler  Form=Parallel  P=20  I=10  D=5  N=100  InitialConditionSource=internal  InitialConditionForIntegrator=0  InitialConditionForFilter=0  ExternalReset=none  LimitOutput=off  UpperSaturationLimit=0.116  LowerSaturationLimit=-0.116  LinearizeAsGain=off  AntiWindupMode=none  Kb=1  TrackingMode=off  Kt=1  PParamMin=[]  PParamMax=[]  IParamMin=[]  IParamMax=[]  DParamMin=[]  DParamMax=[]  NParamMin=[]  NParamMax=[]  KbParamMin=[]  KbParamMax=[]  KtParamMin=[]  KtParamMax=[]  POutMin=[]  POutMax=[]  IOutMin=[]  IOutMax=[]  DOutMin=[]  DOutMax=[]  NOutMin=[]  NOutMax=[]  KbOutMin=[]  KbOutMax=[]  KtOutMin=[]  KtOutMax=[]  IntegratorOutMin=[]  IntegratorOutMax=[]  FilterOutMin=[]  FilterOutMax=[]  SumOutMin=[]  SumOutMax=[]  SumI1OutMin=[]  SumI1OutMax=[]  SumI2OutMin=[]  SumI2OutMax=[]  SumI3OutMin=[]  SumI3OutMax=[]  SumDOutMin=[]  SumDOutMax=[]  SaturationOutMin=[]  SaturationOutMax=[]  IntegratorContinuousStateAttributes=''  IntegratorStateMustResolveToSignalObject=off  IntegratorRTWStateStorageClass=Auto  FilterContinuousStateAttributes=''  FilterStateMustResolveToSignalObject=off  FilterRTWStateStorageClass=Auto  DifferentiatorICPrevScaledInput=0  DifferentiatorOutMin=[]  DifferentiatorOutMax=[]  UseFilter=on
  CrtlPitch : simulink/Continuous/PID Controller  Controller=PD  TimeDomain=Discrete-time  SampleTime=0.001  IntegratorMethod=Forward Euler  FilterMethod=Forward Euler  Form=Parallel  P=2  I=0  D=1  N=100  InitialConditionSource=internal  InitialConditionForIntegrator=0  InitialConditionForFilter=0  ExternalReset=none  LimitOutput=off  UpperSaturationLimit=+Inf  LowerSaturationLimit=0  LinearizeAsGain=off  AntiWindupMode=none  Kb=1  TrackingMode=off  Kt=1  PParamMin=[]  PParamMax=[]  IParamMin=[]  IParamMax=[]  DParamMin=[]  DParamMax=[]  NParamMin=[]  NParamMax=[]  KbParamMin=[]  KbParamMax=[]  KtParamMin=[]  KtParamMax=[]  POutMin=[]  POutMax=[]  IOutMin=[]  IOutMax=[]  DOutMin=[]  DOutMax=[]  NOutMin=[]  NOutMax=[]  KbOutMin=[]  KbOutMax=[]  KtOutMin=[]  KtOutMax=[]  IntegratorOutMin=[]  IntegratorOutMax=[]  FilterOutMin=[]  FilterOutMax=[]  SumOutMin=[]  SumOutMax=[]  SumI1OutMin=[]  SumI1OutMax=[]  SumI2OutMin=[]  SumI2OutMax=[]  SumI3OutMin=[]  SumI3OutMax=[]  SumDOutMin=[]  SumDOutMax=[]  SaturationOutMin=[]  SaturationOutMax=[]  IntegratorContinuousStateAttributes=''  IntegratorStateMustResolveToSignalObject=off  IntegratorRTWStateStorageClass=Auto  FilterContinuousStateAttributes=''  FilterStateMustResolveToSignalObject=off  FilterRTWStateStorageClass=Auto  DifferentiatorICPrevScaledInput=0  DifferentiatorOutMin=[]  DifferentiatorOutMax=[]  UseFilter=on
  CrtlYaw : simulink/Continuous/PID Controller  Controller=PD  TimeDomain=Discrete-time  SampleTime=0.001  IntegratorMethod=Forward Euler  FilterMethod=Forward Euler  Form=Parallel  P=0.05  I=1  D=0.01  N=100  InitialConditionSource=internal  InitialConditionForIntegrator=0  InitialConditionForFilter=0  ExternalReset=none  LimitOutput=off  UpperSaturationLimit=0.01  LowerSaturationLimit=-0.01  LinearizeAsGain=off  AntiWindupMode=none  Kb=1  TrackingMode=off  Kt=1  PParamMin=[]  PParamMax=[]  IParamMin=[]  IParamMax=[]  DParamMin=[]  DParamMax=[]  NParamMin=[]  NParamMax=[]  KbParamMin=[]  KbParamMax=[]  KtParamMin=[]  KtParamMax=[]  POutMin=[]  POutMax=[]  IOutMin=[]  IOutMax=[]  DOutMin=[]  DOutMax=[]  NOutMin=[]  NOutMax=[]  KbOutMin=[]  KbOutMax=[]  KtOutMin=[]  KtOutMax=[]  IntegratorOutMin=[]  IntegratorOutMax=[]  FilterOutMin=[]  FilterOutMax=[]  SumOutMin=[]  SumOutMax=[]  SumI1OutMin=[]  SumI1OutMax=[]  SumI2OutMin=[]  SumI2OutMax=[]  SumI3OutMin=[]  SumI3OutMax=[]  SumDOutMin=[]  SumDOutMax=[]  SaturationOutMin=[]  SaturationOutMax=[]  IntegratorContinuousStateAttributes=''  IntegratorStateMustResolveToSignalObject=off  IntegratorRTWStateStorageClass=Auto  FilterContinuousStateAttributes=''  FilterStateMustResolveToSignalObject=off  FilterRTWStateStorageClass=Auto  DifferentiatorICPrevScaledInput=0  DifferentiatorOutMin=[]  DifferentiatorOutMax=[]  UseFilter=on
  CtrlRoll : simulink/Continuous/PID Controller  Controller=PD  TimeDomain=Discrete-time  SampleTime=0.001  IntegratorMethod=Forward Euler  FilterMethod=Forward Euler  Form=Parallel  P=2  I=0  D=1  N=100  InitialConditionSource=internal  InitialConditionForIntegrator=0  InitialConditionForFilter=0  ExternalReset=none  LimitOutput=off  UpperSaturationLimit=+Inf  LowerSaturationLimit=0  LinearizeAsGain=off  AntiWindupMode=none  Kb=1  TrackingMode=off  Kt=1  PParamMin=[]  PParamMax=[]  IParamMin=[]  IParamMax=[]  DParamMin=[]  DParamMax=[]  NParamMin=[]  NParamMax=[]  KbParamMin=[]  KbParamMax=[]  KtParamMin=[]  KtParamMax=[]  POutMin=[]  POutMax=[]  IOutMin=[]  IOutMax=[]  DOutMin=[]  DOutMax=[]  NOutMin=[]  NOutMax=[]  KbOutMin=[]  KbOutMax=[]  KtOutMin=[]  KtOutMax=[]  IntegratorOutMin=[]  IntegratorOutMax=[]  FilterOutMin=[]  FilterOutMax=[]  SumOutMin=[]  SumOutMax=[]  SumI1OutMin=[]  SumI1OutMax=[]  SumI2OutMin=[]  SumI2OutMax=[]  SumI3OutMin=[]  SumI3OutMax=[]  SumDOutMin=[]  SumDOutMax=[]  SaturationOutMin=[]  SaturationOutMax=[]  IntegratorContinuousStateAttributes=''  IntegratorStateMustResolveToSignalObject=off  IntegratorRTWStateStorageClass=Auto  FilterContinuousStateAttributes=''  FilterStateMustResolveToSignalObject=off  FilterRTWStateStorageClass=Auto  DifferentiatorICPrevScaledInput=0  DifferentiatorOutMin=[]  DifferentiatorOutMax=[]  UseFilter=on
  Gain : Gain  Gain=0.8
  Gain1 : Gain  Gain=0.1
  Gain2 : Gain  Gain=-0.1
  Gain3 : Gain  Gain=0.1
  Gain4 : Gain  Gain=-0.1
  Gain5 : Gain  Gain=0.1
  Gain6 : Gain  Gain=-0.1
  Pitch Cmd : simulink/Discontinuities/Saturation Dynamic  OutMin=[]  OutMax=[]  OutDataTypeStr=Inherit: Same as second input  OutDataType=fixdt(1, 16)  OutScaling=2^-10  DoSatur=off
      settings: LockScale=on
  Ref_Spd_Min : Constant  Value=0
  Roll Cmd : simulink/Discontinuities/Saturation Dynamic  OutMin=[]  OutMax=[]  OutDataTypeStr=Inherit: Same as second input  OutDataType=fixdt(1, 16)  OutScaling=2^-10  DoSatur=off
      settings: LockScale=on
  Saturation Dynamic{,1..3} (4 alike) : simulink/Discontinuities/Saturation Dynamic  OutMin=[]  OutMax=[]  OutDataTypeStr=Inherit: Same as second input  OutDataType=fixdt(1, 16)  OutScaling=2^-10  DoSatur=off
  Sum : Sum  Inputs=|+-+
  Sum2 : Sum  Inputs=|++-
  Sum3 : Sum  Inputs=|+--
  Sum5 : Sum  Inputs=|+++
  Yaw Cmd : simulink/Discontinuities/Saturation Dynamic  OutMin=[]  OutMax=[]  OutDataTypeStr=Inherit: Same as second input  OutDataType=fixdt(1, 16)  OutScaling=2^-10  DoSatur=off
      settings: LockScale=on
  Spd_A : Outport
  Spd_B : Outport  Port=2
  Spd_C : Outport  Port=3
  Spd_D : Outport  Port=4
  wires:
  Saturation Dynamic/1 -> Spd_A/1
  Saturation Dynamic1/1 -> Spd_B/1
  Saturation Dynamic2/1 -> Spd_C/1
  Saturation Dynamic3/1 -> Spd_D/1
  Sum/1 -> Saturation Dynamic/2
  Sum2/1 -> Saturation Dynamic1/2
  Sum5/1 -> Saturation Dynamic2/2
  Sum3/1 -> Saturation Dynamic3/2
  Ref_Spd_Max/1 -> Gain3/1, Gain4/1, Gain5/1, Gain6/1, Gain2/1, Gain1/1, Gain/1, Saturation Dynamic3/1, Saturation Dynamic2/1, Saturation Dynamic1/1, Saturation Dynamic/1
  Ref_Spd_Min/1 -> Saturation Dynamic/3, Saturation Dynamic1/3, Saturation Dynamic2/3, Saturation Dynamic3/3, Altitude Cmd/3
  Err_Alt/1 -> CrtAlt/1
  CrtAlt/1 -> Altitude Cmd/2
  Altitude Cmd/1 -> Sum3/1, Sum5/1, Sum2/1, Sum/1
  Err_Roll/1 -> CtrlRoll/1
  Gain/1 -> Altitude Cmd/1
  CtrlRoll/1 -> Roll Cmd/2
  Gain2/1 -> Roll Cmd/3
  Gain1/1 -> Roll Cmd/1
  Roll Cmd/1 -> Sum2/2, Sum3/2
  Err_Pitch/1 -> CrtlPitch/1
  CrtlPitch/1 -> Pitch Cmd/2
  Gain3/1 -> Pitch Cmd/1
  Gain4/1 -> Pitch Cmd/3
  Pitch Cmd/1 -> Sum/2, Sum5/2
  Err_Yaw/1 -> CrtlYaw/1
  CrtlYaw/1 -> Yaw Cmd/2
  Gain5/1 -> Yaw Cmd/1
  Gain6/1 -> Yaw Cmd/3
  Yaw Cmd/1 -> Sum/3, Sum2/3, Sum5/3, Sum3/3

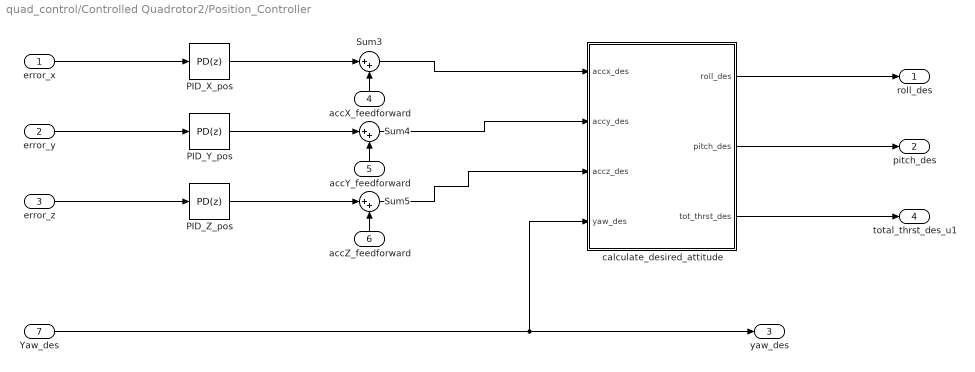
== system quad_control/Controlled Quadrotor2/Position_Controller ==
  error_x : Inport
  error_y : Inport  Port=2
  error_z : Inport  Port=3
  accX_feedforward : Inport  Port=4
  accY_feedforward : Inport  Port=5
  accZ_feedforward : Inport  Port=6
  Yaw_des : Inport  Port=7
  PID_X_pos : simulink/Continuous/PID Controller  Controller=PD  TimeDomain=Discrete-time  SampleTime=0.01  IntegratorMethod=Forward Euler  FilterMethod=Forward Euler  Form=Parallel  P=10  I=1  D=3  N=148.847847480226  InitialConditionSource=internal  InitialConditionForIntegrator=0  InitialConditionForFilter=0  ExternalReset=none  LimitOutput=off  UpperSaturationLimit=inf  LowerSaturationLimit=-inf  LinearizeAsGain=on  AntiWindupMode=none  Kb=1  TrackingMode=off  Kt=1  PParamMin=[]  PParamMax=[]  IParamMin=[]  IParamMax=[]  DParamMin=[]  DParamMax=[]  NParamMin=[]  NParamMax=[]  KbParamMin=[]  KbParamMax=[]  KtParamMin=[]  KtParamMax=[]  POutMin=[]  POutMax=[]  IOutMin=[]  IOutMax=[]  DOutMin=[]  DOutMax=[]  NOutMin=[]  NOutMax=[]  KbOutMin=[]  KbOutMax=[]  KtOutMin=[]  KtOutMax=[]  IntegratorOutMin=[]  IntegratorOutMax=[]  FilterOutMin=[]  FilterOutMax=[]  SumOutMin=[]  SumOutMax=[]  SumI1OutMin=[]  SumI1OutMax=[]  SumI2OutMin=[]  SumI2OutMax=[]  SumI3OutMin=[]  SumI3OutMax=[]  SumDOutMin=[]  SumDOutMax=[]  SaturationOutMin=[]  SaturationOutMax=[]  IntegratorContinuousStateAttributes=''  IntegratorStateMustResolveToSignalObject=off  IntegratorRTWStateStorageClass=Auto  FilterContinuousStateAttributes=''  FilterStateMustResolveToSignalObject=off  FilterRTWStateStorageClass=Auto  DifferentiatorICPrevScaledInput=0  DifferentiatorOutMin=[]  DifferentiatorOutMax=[]  UseFilter=on
  PID_Y_pos : simulink/Continuous/PID Controller  Controller=PD  TimeDomain=Discrete-time  SampleTime=0.01  IntegratorMethod=Forward Euler  FilterMethod=Forward Euler  Form=Parallel  P=10  I=1  D=3  N=100  InitialConditionSource=internal  InitialConditionForIntegrator=0  InitialConditionForFilter=0  ExternalReset=none  LimitOutput=off  UpperSaturationLimit=inf  LowerSaturationLimit=-inf  LinearizeAsGain=on  AntiWindupMode=none  Kb=1  TrackingMode=off  Kt=1  PParamMin=[]  PParamMax=[]  IParamMin=[]  IParamMax=[]  DParamMin=[]  DParamMax=[]  NParamMin=[]  NParamMax=[]  KbParamMin=[]  KbParamMax=[]  KtParamMin=[]  KtParamMax=[]  POutMin=[]  POutMax=[]  IOutMin=[]  IOutMax=[]  DOutMin=[]  DOutMax=[]  NOutMin=[]  NOutMax=[]  KbOutMin=[]  KbOutMax=[]  KtOutMin=[]  KtOutMax=[]  IntegratorOutMin=[]  IntegratorOutMax=[]  FilterOutMin=[]  FilterOutMax=[]  SumOutMin=[]  SumOutMax=[]  SumI1OutMin=[]  SumI1OutMax=[]  SumI2OutMin=[]  SumI2OutMax=[]  SumI3OutMin=[]  SumI3OutMax=[]  SumDOutMin=[]  SumDOutMax=[]  SaturationOutMin=[]  SaturationOutMax=[]  IntegratorContinuousStateAttributes=''  IntegratorStateMustResolveToSignalObject=off  IntegratorRTWStateStorageClass=Auto  FilterContinuousStateAttributes=''  FilterStateMustResolveToSignalObject=off  FilterRTWStateStorageClass=Auto  DifferentiatorICPrevScaledInput=0  DifferentiatorOutMin=[]  DifferentiatorOutMax=[]  UseFilter=on
  PID_Z_pos : simulink/Continuous/PID Controller  Controller=PD  TimeDomain=Discrete-time  SampleTime=0.01  IntegratorMethod=Forward Euler  FilterMethod=Forward Euler  Form=Parallel  P=2  I=10  D=0.001  N=100  InitialConditionSource=internal  InitialConditionForIntegrator=0  InitialConditionForFilter=0  ExternalReset=none  LimitOutput=off  UpperSaturationLimit=inf  LowerSaturationLimit=-inf  LinearizeAsGain=on  AntiWindupMode=none  Kb=1  TrackingMode=off  Kt=1  PParamMin=[]  PParamMax=[]  IParamMin=[]  IParamMax=[]  DParamMin=[]  DParamMax=[]  NParamMin=[]  NParamMax=[]  KbParamMin=[]  KbParamMax=[]  KtParamMin=[]  KtParamMax=[]  POutMin=[]  POutMax=[]  IOutMin=[]  IOutMax=[]  DOutMin=[]  DOutMax=[]  NOutMin=[]  NOutMax=[]  KbOutMin=[]  KbOutMax=[]  KtOutMin=[]  KtOutMax=[]  IntegratorOutMin=[]  IntegratorOutMax=[]  FilterOutMin=[]  FilterOutMax=[]  SumOutMin=[]  SumOutMax=[]  SumI1OutMin=[]  SumI1OutMax=[]  SumI2OutMin=[]  SumI2OutMax=[]  SumI3OutMin=[]  SumI3OutMax=[]  SumDOutMin=[]  SumDOutMax=[]  SaturationOutMin=[]  SaturationOutMax=[]  IntegratorContinuousStateAttributes=''  IntegratorStateMustResolveToSignalObject=off  IntegratorRTWStateStorageClass=Auto  FilterContinuousStateAttributes=''  FilterStateMustResolveToSignalObject=off  FilterRTWStateStorageClass=Auto  DifferentiatorICPrevScaledInput=0  DifferentiatorOutMin=[]  DifferentiatorOutMax=[]  UseFilter=on
  Sum3 : Sum  Inputs=|++
  Sum4 : Sum  Inputs=|++
  Sum5 : Sum  Inputs=|++
  calculate_desired_attitude : MATLAB Function  TreatAsAtomicUnit=on
  roll_des : Outport
  pitch_des : Outport  Port=2
  yaw_des : Outport  Port=3
  total_thrst_des_u1 : Outport  Port=4
  wires:
  PID_Z_pos/1 -> Sum5/1
  PID_Y_pos/1 -> Sum4/1
  accX_feedforward/1 -> Sum3/2
  calculate_desired_attitude/3(tot_thrst_des) -> total_thrst_des_u1/1
  Yaw_des/1 -> calculate_desired_attitude/4(yaw_des), yaw_des/1
  accZ_feedforward/1 -> Sum5/2
  accY_feedforward/1 -> Sum4/2
  Sum4/1 -> calculate_desired_attitude/2(accy_des)
  Sum3/1 -> calculate_desired_attitude/1(accx_des)
  PID_X_pos/1 -> Sum3/1
  Sum5/1 -> calculate_desired_attitude/3(accz_des)
  error_x/1 -> PID_X_pos/1
  error_y/1 -> PID_Y_pos/1
  error_z/1 -> PID_Z_pos/1
  calculate_desired_attitude/1(roll_des) -> roll_des/1
  calculate_desired_attitude/2(pitch_des) -> pitch_des/1
